simulink model "SZAU_lin"  (R2017b)
settings: Solver=VariableStepAuto  StartTime=0.0  StopTime=150  RelTol=1e-3
values from neighbouring files (symbols this model uses):
  A1 = 505    [SZAU_lin.mat]
  a1 = 22    [SZAU_lin.mat]
  a2 = 16    [SZAU_lin.mat]
  C2 = 0.65    [SZAU_lin.mat]
  Fd = 13    [SZAU_lin.mat]
  h10 = 17.87    [SZAU_lin.mat]
settings Model: Creator=Jarzyn  LastModifiedBy=Jarzyn

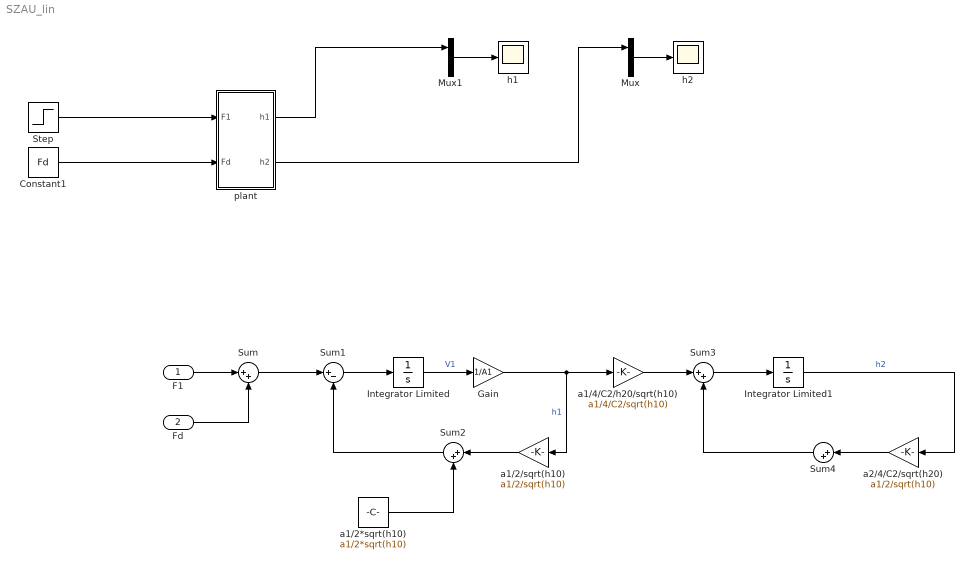
== system SZAU_lin ==
  F1 : Inport
  Fd : Inport  Port=2
  Constant1 : Constant  Value=Fd
  Gain : Gain  Gain=1/A1
  Integrator Limited : Integrator  LimitOutput=on  UpperSaturationLimit=1  LowerSaturationLimit=0
  Integrator Limited1 : Integrator  LimitOutput=on  UpperSaturationLimit=1  LowerSaturationLimit=0
  Mux : Mux  Inputs=2
  Mux1 : Mux  Inputs=2
  Step : Step  Time=0  After=10  SampleTime=1
  Sum{,2..4} (4 alike) : Sum  Inputs=|++
  Sum1 : Sum  Inputs=|+-
  a1/2*sqrt(h10) : Constant  Value=a1/2*sqrt(h10)
  a1/2/sqrt(h10) : Gain  Gain=a1/2/sqrt(h10)
  a1/4/C2/h20/sqrt(h10) : Gain  Gain=a1/4/C2/sqrt(h10)
  a2/4/C2/sqrt(h20) : Gain  Gain=a1/2/sqrt(h10)
  h1 : Scope
  h2 : Scope
  plant : Subsystem
  wires:
  plant/2(h2) -> Mux/1
  Mux/1 -> h2/1
  plant/1(h1) -> Mux1/1
  Mux1/1 -> h1/1
  Step/1 -> plant/1(F1)
  Constant1/1 -> plant/2(Fd)
  F1/1 -> Sum/1
  Fd/1 -> Sum/2
  Sum/1 -> Sum1/1
  Sum1/1 -> Integrator Limited/1
  Integrator Limited/1 -> Gain/1  "V1"
  Gain/1 -> a1/4/C2/h20/sqrt(h10)/1, a1/2/sqrt(h10)/1  "h1"
  Sum2/1 -> Sum1/2
  a1/2*sqrt(h10)/1 -> Sum2/2
  a1/2/sqrt(h10)/1 -> Sum2/1
  a1/4/C2/h20/sqrt(h10)/1 -> Sum3/1
  Sum3/1 -> Integrator Limited1/1
  ? -> Sum4/2
  Sum4/1 -> Sum3/2
  Integrator Limited1/1 -> a2/4/C2/sqrt(h20)/1  "h2"
  a2/4/C2/sqrt(h20)/1 -> Sum4/1

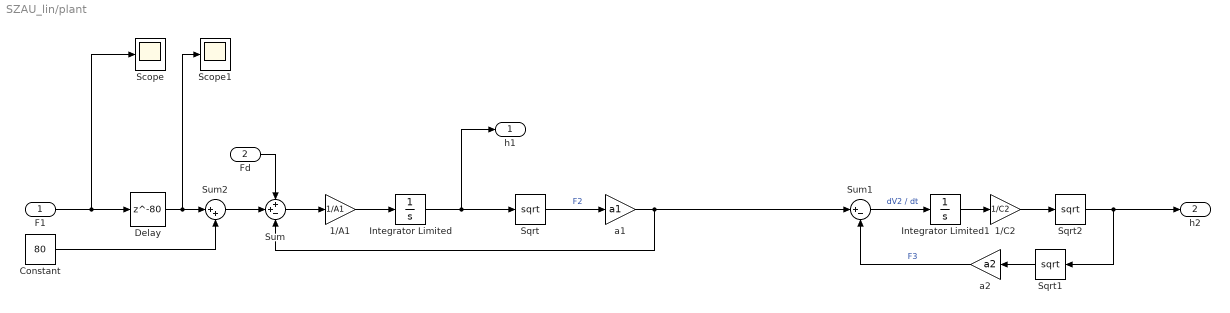
== system SZAU_lin/plant ==
  F1 : Inport
  Fd : Inport  Port=2
  1/A1 : Gain  Gain=1/A1
  1/C2 : Gain  Gain=1/C2
  Constant : Constant  Value=80
  Delay : Delay  DelayLength=80  InitialCondition=0
  Integrator Limited : Integrator  InitialCondition=h10  LimitOutput=on  LowerSaturationLimit=0
  Integrator Limited1 : Integrator  InitialCondition=0.65*33.7852^2  LimitOutput=on  LowerSaturationLimit=0
  Scope : Scope
  Scope1 : Scope
  Sqrt : Sqrt  SaturateOnIntegerOverflow=on
  Sqrt1 : Sqrt  SaturateOnIntegerOverflow=on
  Sqrt2 : Sqrt  SaturateOnIntegerOverflow=on
  Sum : Sum  Inputs=++-
  Sum1 : Sum  Inputs=|+-
  Sum2 : Sum  Inputs=|++
  a1 : Gain  Gain=a1
  a2 : Gain  Gain=a2
  h1 : Outport
  h2 : Outport  Port=2
  wires:
  F1/1 -> Scope/1, Delay/1
  Sqrt1/1 -> a2/1
  Fd/1 -> Sum/1
  Sum/1 -> 1/A1/1
  1/A1/1 -> Integrator Limited/1
  Sqrt2/1 -> Sqrt1/1, h2/1
  a2/1 -> Sum1/2  "F3"
  Integrator Limited/1 -> h1/1, Sqrt/1
  Sqrt/1 -> a1/1  "F2"
  a1/1 -> Sum/3, Sum1/1
  Integrator Limited1/1 -> 1/C2/1
  Delay/1 -> Scope1/1, Sum2/1
  Sum2/1 -> Sum/2
  1/C2/1 -> Sqrt2/1
  Sum1/1 -> Integrator Limited1/1  "dV2 / dt"
  Constant/1 -> Sum2/2
